simulink model "SVL_VV_schema"  (R2018b)
settings: Solver=VariableStepAuto  StartTime=0.0  StopTime=10  RelTol=1e-3
undefined symbols (not defined in the file): ziad
settings Model: Creator=Marek  LastModifiedBy=Marek

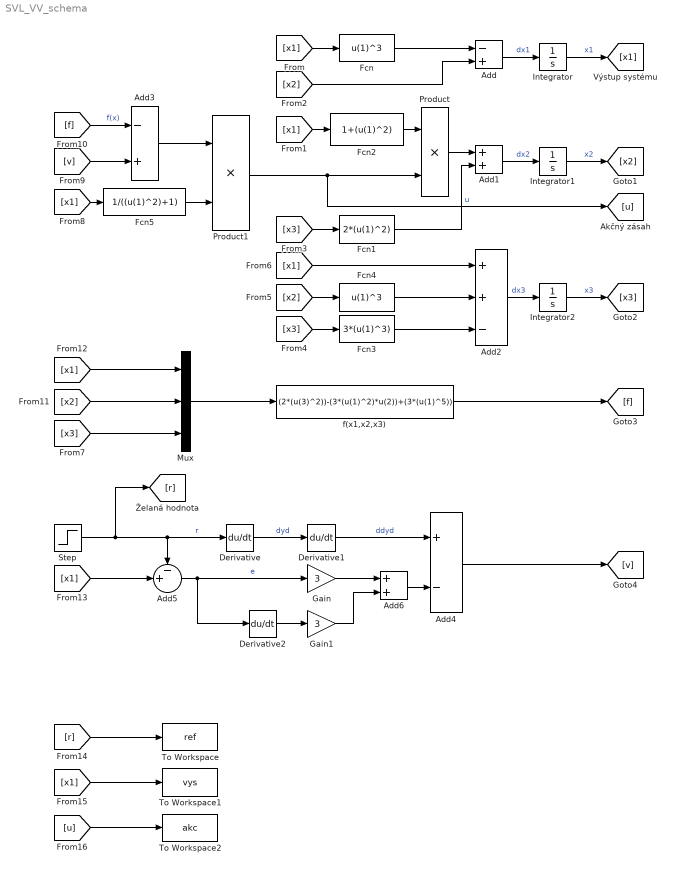
== system SVL_VV_schema ==
  Add : Sum  Inputs=-+
  Add1 : Sum
  Add2 : Sum  Inputs=++-
  Add3 : Sum  Inputs=-+
  Add4 : Sum  Inputs=+-
  Add5 : Sum  Inputs=-+|
  Add6 : Sum
  Derivative : Derivative
  Derivative1 : Derivative
  Derivative2 : Derivative
  Fcn : Fcn  Expr=u(1)^3
  Fcn1 : Fcn  Expr=2*(u(1)^2)
  Fcn2 : Fcn  Expr=1+(u(1)^2)
  Fcn3 : Fcn  Expr=3*(u(1)^3)
  Fcn4 : Fcn  Expr=u(1)^3
  Fcn5 : Fcn  Expr=1/((u(1)^2)+1)
  Gain : Gain  Gain=3
  Gain1 : Gain  Gain=3
  Integrator : Integrator
  Integrator1 : Integrator
  Integrator2 : Integrator
  Mux : Mux  Inputs=3
  Product : Product
  Product1 : Product
  Step : Step  Time=0  After=ziad  SampleTime=0
  To Workspace : ToWorkspace  VariableName=ref  SaveFormat=Timeseries  SampleTime=-1
  To Workspace1 : ToWorkspace  VariableName=vys  SaveFormat=Timeseries  SampleTime=-1
  To Workspace2 : ToWorkspace  VariableName=akc  SaveFormat=Timeseries  SampleTime=-1
  f(x1,x2,x3) : Fcn  Expr=(2*(u(3)^2))-(3*(u(1)^2)*u(2))+(3*(u(1)^5))
  wires:
  Integrator/1 -> [x1]  "x1"
  Integrator2/1 -> [x3]  "x3"
  Add/1 -> Integrator/1  "dx1"
  Fcn/1 -> Add/1
  Add1/1 -> Integrator1/1  "dx2"
  Fcn1/1 -> Add1/2
  Product/1 -> Add1/1
  Fcn2/1 -> Product/1
  Product1/1 -> [u], Product/2  "u"
  Add2/1 -> Integrator2/1  "dx3"
  Fcn3/1 -> Add2/3
  [x1] -> Fcn/1
  [x1] -> Fcn2/1
  [x2] -> Add/2
  Integrator1/1 -> [x2]  "x2"
  [x3] -> Fcn1/1
  [x3] -> Fcn3/1
  [x2] -> Fcn4/1
  Fcn4/1 -> Add2/2
  [x1] -> Add2/1
  Fcn5/1 -> Product1/2
  [x1] -> Fcn5/1
  Add3/1 -> Product1/1
  [v] -> Add3/2
  [f] -> Add3/1  "f(x)"
  [x3] -> Mux/3
  [x1] -> Mux/1
  [x2] -> Mux/2
  Mux/1 -> f(x1,x2,x3)/1
  f(x1,x2,x3)/1 -> [f]
  Step/1 -> Derivative/1, Add5/1, [r]  "r"
  Derivative/1 -> Derivative1/1  "dyd"
  Derivative1/1 -> Add4/1  "ddyd"
  Add4/1 -> [v]
  [x1] -> Add5/2
  Add5/1 -> Gain/1, Derivative2/1  "e"
  Gain/1 -> Add6/1
  Add6/1 -> Add4/2
  Derivative2/1 -> Gain1/1
  Gain1/1 -> Add6/2
  [r] -> To Workspace/1
  [x1] -> To Workspace1/1
  [u] -> To Workspace2/1
